simulink model "MeresHoltidoMotrokcosim"  (R2013b)
settings: Solver=FixedStepDiscrete  SolverMode=SingleTasking  StartTime=0.0  StopTime=inf  FixedStep=1  RelTol=1e-3
undefined symbols (not defined in the file or in its folder): A, N
libraries: xbsIndex_r4 x2, simulink x2, JTAGRuntimeCosim_r4 x1
settings Model: Creator=laca  LastModifiedBy=laca
settings DebuggingCC: MultiTaskDSMMsg=warning  MultiTaskCondExecSysMsg=none  FcnCallInpInsideContextMsg=EnableAllAsWarning
settings RTWCC: IncludeERTFirstTime=on

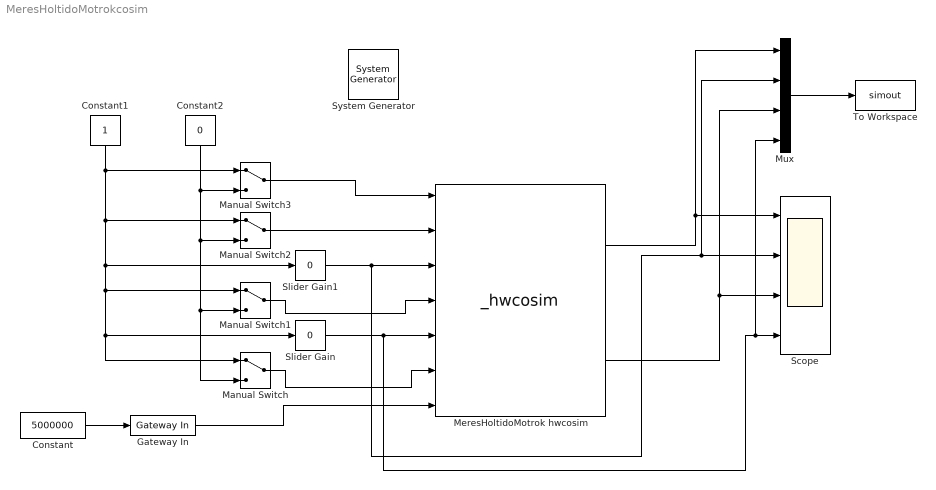
== system MeresHoltidoMotrokcosim ==
  " System Generator" : xbsIndex_r4/ System Generator  Tag=genX  xilinxfamily=spartan3e  part=xc3s500e  speed=-4  package=pq208  synthesis_tool=XST  clock_wrapper=Clock Enables  directory=./netlist  proj_type=Project Navigator  Synth_file=XST Defaults  Impl_file=ISE Defaults  testbench=off  simulink_period=1  sysclk_period=20  dcm_input_clock_period=10  incr_netlist=off  trim_vbits=Everywhere in SubSystem  dbl_ovrd=According to Block Masks  core_generation=According to Block Masks  run_coregen=off  deprecated_control=off  eval_field=0  block_type=sysgen
  Constant : Constant  Value=5000000
  Constant1 : Constant
  Constant2 : Constant  Value=0
  Gateway In : xbsIndex_r4/Gateway In  gui_display_data_type=Fixed-point  arith_type=Unsigned  n_bits=32  bin_pt=0  preci_type=Single  exp_width=8  frac_width=24  quantization="Round  (unbiased: +/- Inf)"  overflow=Saturate  period=1  dbl_ovrd=off  timing_constraint=None  locs_specified=off  LOCs={}  UseAsADC=off  ADCChannel='1'  inherit_from_input=off  hdl_port=on  block_type=gatewayin
  Manual Switch{,1..3} (4 alike) : ManualSwitch
  MeresHoltidoMotrok hwcosim : JTAGRuntimeCosim_r4/_hwcosim  clkSrc=Free Running  hasCombinationalPath=off  bitfileName=C:\Diak\gl\SPARTAN3E500K_slave\SystemGenrator\SebessegEsPozicio\netlist\meresholtidomotrok_cw.bit  skipConfig=off  cable=Auto Detect  speed=N/A  cablePort=N/A  cableLocation=Local  shareCable=off  enable_codebug=on  design_xtable=|  engineDll=JTAGCosimEngine.dll  cableWaitTime=10  bscanPos=1  IRLengths=[6,8]  useWaitBox=1  hasBufgmux=on  Scheme=Cosim  useCmdProc=1  hasProc=0  useImpact=0  printLogFile=0  block_type=jtagcosim
      | {
      |   'clkWrapper' => 'meresholtidomotrok_cw',
      |   'clocksGcd' => undef,
      |   'device' => 'xc3s500e-4pq208',
      |   'ports' => {
      |     'csereposdir' => {
      |       'bd_port_index' => 0,
      |       'direction' => 'in',
      |       'icon_text' => 'cserePosdir',
      |       'period' => 1,
      |       'sim_pause_trigger' => false,
      |       'type' => 'Bool',
      |       'width' => 1,
      |     },
      |     'cseresebdir' => {
      |       'bd_port_index' => 1,
      |       'direction' => 'in',
      |       'icon_text' => 'csereSebdir',
      |       'period' => 1,
      |       'sim_pause_trigger' => false,
      |       'type' => 'Bool',
      |       'width' => 1,
      |     },
      |     'pos' => {
      |       'bd_port_index' => 2,
      |       'direction' => 'in',
      |       'icon_text' => 'pos',
      |       'period' => 1,
      |       'sim_pause_trigger' => false,
      |       'type' => 'Fix_17_0',
      |       'width' => 17,
      |     },
      |     'pos_en' => {
      |       'bd_port_index' => 3,
      |       'direction' => 'in',
      |       'icon_text' => 'pos en',
      |       'period' => 1,
      |       'sim_pause_trigger' => false,
      |       'type' => 'Bool',
      |       'width' => 1,
      |     },
      |     'position' => {
      |       'bd_port_index' => 0,
      |       'direction' => 'out',
      |       'icon_text' => 'Position',
      |       'period' => 1,
      |       'sim_pause_trigger' => false,
      |       'type' => 'Fix_16_0',
      |       'width' => 16,
      |     },
      |     'seb' => {
      |       'bd_port_index' => 4,
      |       'direction' => 'in',
      |       'icon_text' => 'seb',
      |       'period' => 1,
      |       'sim_pause_trigger' => false,
      |       'type' => 'Fix_17_0',
      |       'width' => 17,
      |     },
      |     'seben' => {
      |       'bd_port_index' => 5,
      |       'direction' => 'in',
      |       'icon_text' => 'seben',
      |       'period' => 1,
      |       'sim_pause_trigger' => false,
      |       'type' => 'Bool',
      |       'width' => 1,
      |     },
      |     'sebesseg' => {
      |       'bd_port_index' => 1,
      |       'direction' => 'out',
      |       'icon_text' => 'sebesseg',
      |       'period' => 1,
      |       'sim_pause_trigger' => false,
      |       'type' => 'Fix_16_0',
      |       'width' => 16,
      |     },
      |     'tsreg' => {
      |       'bd_port_index' => 6,
      |       'direction' => 'in',
      |       'icon_text' => 'Tsreg',
      |       'period' => 1,
      |       'sim_pause_trigger' => false,
      |       'type' => 'UFix_32_0',
      |       'width' => 32,
      |     },
      |   },
      |   'shared_memories' => {},
      | }
  Mux : Mux
  Scope : Scope  NumInputPorts=4
      settings: YMin=-20~-1~-1~1  YMax=-20~1~1~1
  Slider Gain : simulink/Math Operations/Slider Gain  low=-65000  gain=0  high=65000
  Slider Gain1 : simulink/Math Operations/Slider Gain  low=-65000  gain=0  high=65000
  To Workspace : ToWorkspace  VariableName=simout  SampleTime=-1  SaveFormat=Timeseries
  wires:
  Constant/1 -> Gateway In/1
  Manual Switch/1 -> MeresHoltidoMotrok hwcosim/6
  Manual Switch1/1 -> MeresHoltidoMotrok hwcosim/4
  Slider Gain1/1 -> MeresHoltidoMotrok hwcosim/3, Mux/2, Scope/2
  Manual Switch2/1 -> MeresHoltidoMotrok hwcosim/2
  Manual Switch3/1 -> MeresHoltidoMotrok hwcosim/1
  Constant2/1 -> Manual Switch3/2, Manual Switch2/2, Manual Switch1/2, Manual Switch/2
  Constant1/1 -> Manual Switch3/1, Manual Switch2/1, Slider Gain1/1, Manual Switch1/1, Slider Gain/1, Manual Switch/1
  MeresHoltidoMotrok hwcosim/1 -> Mux/1, Scope/1
  MeresHoltidoMotrok hwcosim/2 -> Mux/3, Scope/3
  Slider Gain/1 -> MeresHoltidoMotrok hwcosim/5, Mux/4, Scope/4
  Mux/1 -> To Workspace/1
  Gateway In/1 -> MeresHoltidoMotrok hwcosim/7
